simulink model "laba4_MSK"  (Simulink 7.5)
settings: Solver=ode45  StartTime=0.0  StopTime=10.0  RelTol=1e-3
undefined symbols (not defined in the file): Fs, get, sided, Two
libraries: dspbuff3 x4, commsequence2 x1, commseqgen2 x1, dspspect3 x1, simulink x1, dspsnks4 x1, commutil2 x1
settings Model: Creator=Lenovo  LastModifiedBy=Lenovo

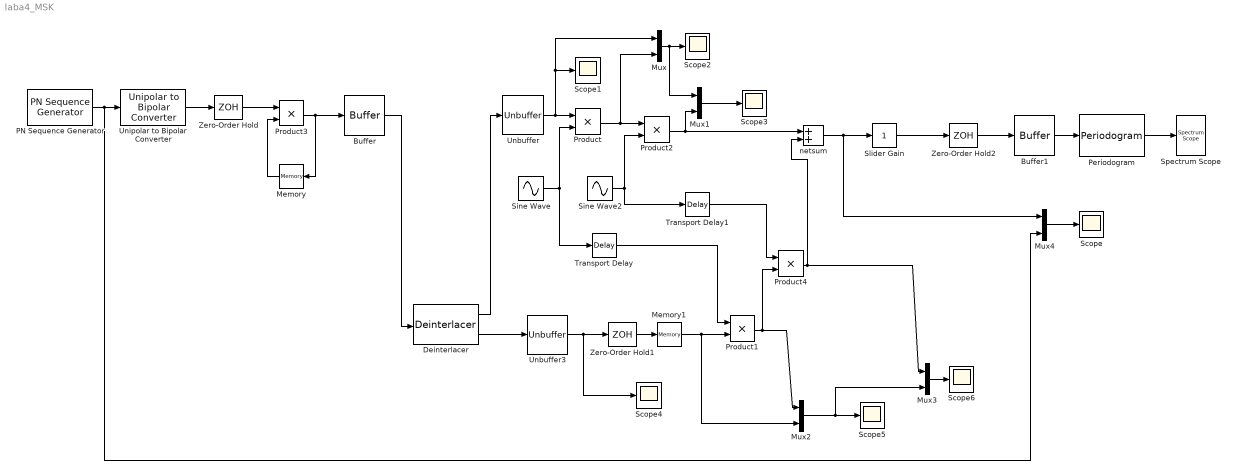
== system laba4_MSK ==
  Buffer : dspbuff3/Buffer  N=2  V=0  ic=0
  Buffer1 : dspbuff3/Buffer  N=64  V=0  ic=0
  Deinterlacer : commsequence2/Deinterlacer
  Memory : Memory  X0=1  InheritSampleTime=on
  Memory1 : Memory  InheritSampleTime=on
  Mux{,1..4} (5 alike) : Mux  Inputs=2
  PN Sequence Generator : commseqgen2/PN Sequence Generator  poly=[1 0 0 0 0 1 1]  ini_sta=[0 0 0 0 0 1]  outBitMaskSource=Dialog parameter  shift=0  Ts=1/1200  frameBased=off  sampPerFrame=1  reset=off  bitPackedOutputs=off  outDataType=double  numPackedBits=8  bitPackDataSigned=off  bitPackedOutDType=double
  Periodogram : dspspect3/Periodogram  SystemSampleTime=-1  measurement=Power spectral density  wintype=Hamming  Rs=50  beta=5  winsamp=Symmetric  inheritFFT=off  fftsize=256  navg=4  inheritTs=on  Ts=1
  Product{,1..4} (5 alike) : Product  OutDataType=fixdt(1, 16)  OutScaling=2^0  RndMeth=Zero
  Scope{,1..6} (7 alike) : Scope
      Scope settings: SaveName=ScopeData6
      Scope2 settings: SaveName=ScopeData2
      Scope3 settings: SaveName=ScopeData3
      Scope5 settings: SaveName=ScopeData4
      Scope6 settings: SaveName=ScopeData5
  Sine Wave : Sin  Amplitude=1  Bias=0  Frequency=600*pi  Phase=-pi  Samples=10  SampleTime=0  Offset=0
  Sine Wave2 : Sin  Amplitude=1  Bias=0  Frequency=76000*pi  Phase=0  Samples=10  SampleTime=0  Offset=0
  Slider Gain : simulink/Math Operations/Slider Gain  SystemSampleTime=-1  low=0  gain=1  high=2
  Spectrum Scope : dspsnks4/Spectrum Scope  DialogController=dspdialog.SpectrumScope  DialogControllerArgs=DataTag0  SystemSampleTime=-1  ScopeProperties=on  Domain=Frequency  HorizSpan=1  UseBuffer=off  BufferSize=128  Overlap=64  inpFftLenInherit=off  FFTlength=128  numAvg=2  DisplayProperties=off  AxisGrid=on  Memory=off  FrameNumber=on  AxisLegend=off  AxisZoom=off  OpenScopeAtSimStart=on  OpenScopeImmediately=off  FigPos=get(0,'defaultfigureposition')  AxisProperties=off  XUnits=Hertz  XRange=Two-sided ((-Fs/2...Fs/2])  XDisplay=0  InheritXIncr=on  XIncr=1.0  XLabel=Samples  XLimit=Auto  YUnits=dBW/Hertz  XMax=1  XMin=0  YLabel=Magnitude-squared, dB  LineProperties=off  wintypeSpecScope=Hann  RsSpecScope=50  betaSpecScope=5  winsampSpecScope=Periodic  XAxisParamsVer=6.9
      settings: YMin=-10  YMax=10
  Transport Delay : TransportDelay  DelayTime=1/1200
  Transport Delay1 : TransportDelay  DelayTime=3/38000/4
  Unbuffer : dspbuff3/Unbuffer  ic=0
  Unbuffer3 : dspbuff3/Unbuffer  ic=0
  Unipolar to Bipolar Converter : commutil2/Unipolar to Bipolar Converter  SystemSampleTime=-1  M=2  polarity=Positive  dataType=Inherit via internal rule
  Zero-Order Hold : ZeroOrderHold  SampleTime=1/1200
  Zero-Order Hold1 : ZeroOrderHold  SampleTime=1/1200
  Zero-Order Hold2 : ZeroOrderHold  SampleTime=1/4000/3
  netsum : Sum  Inputs=2  OutDataType=sfix(16)  OutScaling=2^0  SaturateOnIntegerOverflow=on  InputSameDT=on  OutDataTypeStr=Inherit: Same as first input
  wires:
  PN Sequence Generator/1 -> Unipolar to Bipolar Converter/1, Mux4/2
  Unipolar to Bipolar Converter/1 -> Zero-Order Hold/1
  Zero-Order Hold/1 -> Product3/1
  Product3/1 -> Buffer/1, Memory/1
  Buffer/1 -> Deinterlacer/1
  Deinterlacer/1 -> Unbuffer/1
  Deinterlacer/2 -> Unbuffer3/1
  Unbuffer3/1 -> Zero-Order Hold1/1, Scope4/1
  Zero-Order Hold1/1 -> Memory1/1
  Unbuffer/1 -> Product/1, Mux/1, Scope1/1
  Memory/1 -> Product3/2
  Product/1 -> Product2/1, Mux/2
  Sine Wave/1 -> Product/2, Transport Delay/1
  Mux/1 -> Scope2/1, Mux1/1
  Memory1/1 -> Product1/2, Mux2/2
  Sine Wave2/1 -> Product2/2, Transport Delay1/1
  Product2/1 -> netsum/1, Mux1/2
  Mux1/1 -> Scope3/1
  netsum/1 -> Slider Gain/1, Mux4/1
  Slider Gain/1 -> Zero-Order Hold2/1
  Zero-Order Hold2/1 -> Buffer1/1
  Buffer1/1 -> Periodogram/1
  Periodogram/1 -> Spectrum Scope/1
  Product4/1 -> netsum/2, Mux3/1
  Transport Delay/1 -> Product1/1
  Transport Delay1/1 -> Product4/1
  Product1/1 -> Product4/2, Mux2/1
  Mux4/1 -> Scope/1
  Mux3/1 -> Scope6/1
  Mux2/1 -> Scope5/1, Mux3/2
